simulink model "lab10"  (R2024a)
settings: Solver=VariableStepAuto  StartTime=0.0  StopTime=100  RelTol=1e-3  EnableMultiTasking=on
model workspace (MAT data in the model file):
  GGwp = 5
undefined symbols (not defined in the file): m, n
libraries: simulink x2, spsMonostableLib x1, commrandsrc3 x1
settings Model: SimulationMode=accelerator  Creator=The MathWorks, Inc.  LastModifiedBy=user
settings SolverCC: AlgebraicLoopSolver=TrustRegion
settings DataIOCC: LimitDataPoints=on  SaveFormat=Array  ReturnWorkspaceOutputs=off
settings OptimizationCC: LifeSpan=inf
settings DebuggingCC: UnconnectedInputMsg=warning  UnconnectedOutputMsg=warning  UnconnectedLineMsg=warning  AllowSymbolicDim=off  SFUnexpectedBacktrackingDiag=warning  SFNoUnconditionalDefaultTransitionDiag=warning  SFExecutionAtInitializationDiag=none  ArithmeticOperatorsInVariantConditions=warning
settings ModelReferenceCC: EnableRefExpFcnMdlSchedulingChecks=on  PropagateSignalLabelsOutOfModel=off
settings SFSimCC: SimUseLocalCustomCode=off  CustomCodeUndefinedFunction=UseInterfaceOnly
settings RTWCC: RTWUseLocalCustomCode=off  GPUComputeCapability=3.5  DLArmComputeVersion=19.05
settings CodeAppCC: StateflowObjectComments=on
settings GRTTargetCC: TargetLangStandard=C89/C90 (ANSI)
settings ConfigComp: CovMetricSettings=dw  CovSaveCumulativeToWorkspaceVar=on  CovSaveSingleToWorkspaceVar=on  CovExternalEMLEnable=off  CovSFcnEnable=off

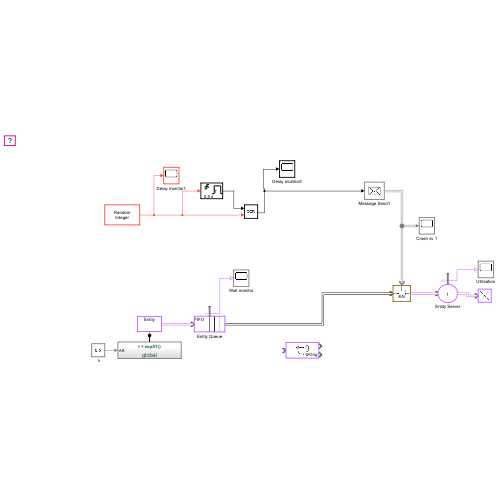
[thumbnail: Simulink's stored preview of the top-level diagram]
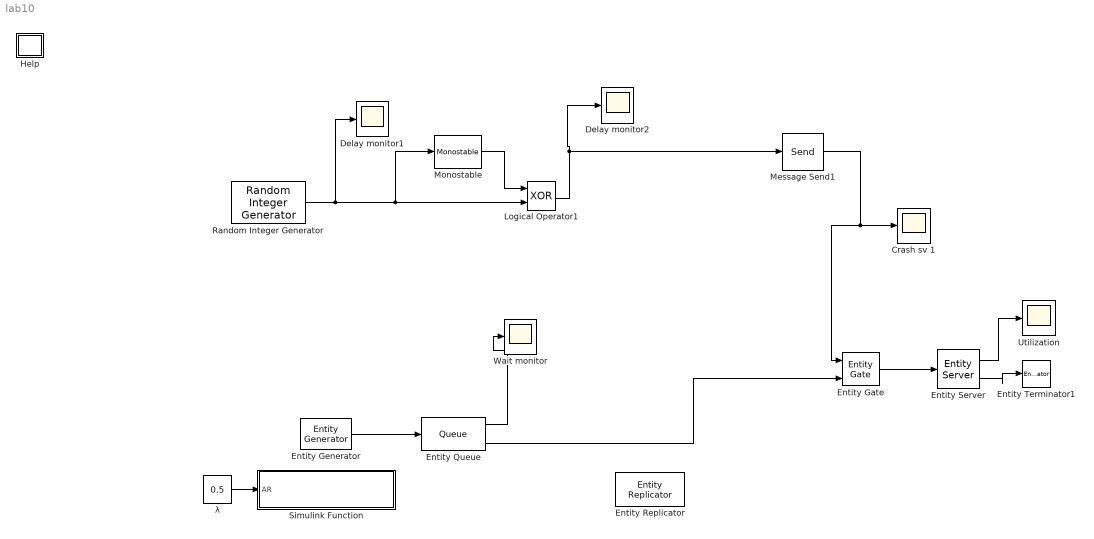
== system lab10 ==
  " λ" : Constant  Value=0.5  SampleTime=-1
  Crash sv 1 : Scope
  Delay monitor1 : Scope
  Delay monitor2 : Scope
  Entity Gate : EntityGate  InputPortMessageModes=m,m  OutputPortMessageModes=m
  Entity Generator : EntityGenerator  OutputPortMessageModes=m  TimeSource=MATLAB action  IntergenerationTimeAction=dt = expAT();  AttributeName=entity  AttributeInitialValue=0  EntityType=Structured  EntityTypeName=Entity
  Entity Queue : Queue  InputPortMessageModes=m  OutputPortMessageModes=n,m  Capacity=inf  AverageWait=on
      settings: OutputPortMap=o2,o5
  Entity Replicator : EntityReplicator  InputPortMessageModes=m  OutputPortMessageModes=m,m
  Entity Server : EntityServer  InputPortMessageModes=m  OutputPortMessageModes=n,m  Capacity=1  Utilization=on
      settings: OutputPortMap=o5,o9
  Entity Terminator1 : EntityTerminator  InputPortMessageModes=m
  Help : Subsystem
      settings: OpenFcn=showExample('simevents/MM1QueuingSysExample');
      mask Display: disp('?')
  Logical Operator1 : Logic  Operator=XOR  AllPortsSameDT=off  OutDataTypeStr=boolean
  Message Send1 : Send  OutputPortMessageModes=m
  Monostable : spsMonostableLib/Monostable  EdgeDetect=Rising  PulseDuration=0.5  ic=1  Ts=0
      settings: LibrarySourceBlock=sps_lib/Control/Monostable
  Random Integer Generator : commrandsrc3/Random Integer Generator  SetSize=2  SeedSource=Parameter  Seed=0  SampleTime=1  SamplesPerFrame=1  OutputDataType=boolean  SimulateUsing=Interpreted execution
  Simulink Function : Subsystem  TreatAsAtomicUnit=on
  Utilization : Scope
  Wait monitor : Scope
  wires:
  " λ"/1 -> Simulink Function/1(AR)
  Entity Gate/1 -> Entity Server/1
  Entity Generator/1 -> Entity Queue/1
  Message Send1/1 -> Entity Gate/1, Crash sv 1/1
  Logical Operator1/1 -> Delay monitor2/1, Message Send1/1
  Entity Queue/1 -> Wait monitor/1
  Entity Server/2 -> Entity Terminator1/1
  Random Integer Generator/1 -> Delay monitor1/1, Monostable/1, Logical Operator1/2
  Entity Server/1 -> Utilization/1
  Monostable/1 -> Logical Operator1/1
  Entity Queue/2 -> Entity Gate/2

== system lab10/Help ==

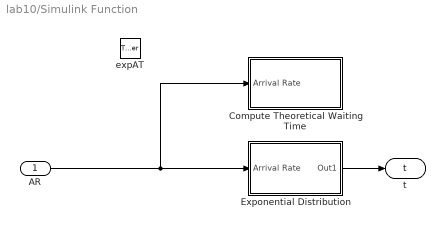
== system lab10/Simulink Function ==
  AR : Inport
  expAT : TriggerPort  TriggerType=function-call  IsSimulinkFunction=on  FunctionName=expAT  VariantControl=Variant
  Compute Theoretical Waiting Time : Subsystem
  Exponential Distribution : Subsystem
  t : ArgOut  DisableCoverage=on  ArgumentName=t
  wires:
  AR/1 -> Compute Theoretical Waiting Time/1(Arrival Rate), Exponential Distribution/1(Arrival Rate)
  Exponential Distribution/1(Out1) -> t/1

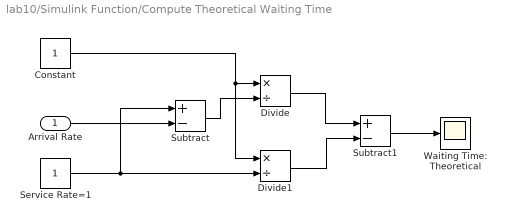
== system lab10/Simulink Function/Compute Theoretical Waiting Time ==
  Arrival Rate : Inport
  Constant : Constant
  Divide : Product  Inputs=*/
  Divide1 : Product  Inputs=*/
  Service Rate=1 : Constant
  Subtract : Sum  Inputs=+-
  Subtract1 : Sum  Inputs=+-
  Waiting Time: Theoretical : Scope
  wires:
  Arrival Rate/1 -> Subtract/2
  Subtract1/1 -> Waiting Time: Theoretical/1
  Divide1/1 -> Subtract1/2
  Divide/1 -> Subtract1/1
  Subtract/1 -> Divide/2
  Constant/1 -> Divide1/1, Divide/1
  Service Rate=1/1 -> Subtract/1, Divide1/2

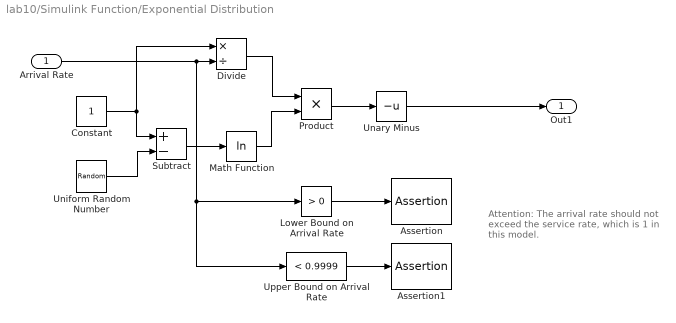
== system lab10/Simulink Function/Exponential Distribution ==
  note: Attention: The arrival rate
      | should not exceed the service
      | rate, which is 1 in this model.
  Arrival Rate : Inport
  Assertion : Assertion
  Assertion1 : Assertion
  Constant : Constant
  Divide : Product  Inputs=*/
  Lower Bound on Arrival Rate : simulink/Logic and Bit Operations/Compare To Constant  relop=>  const=0  OutDataTypeStr=uint8  ZeroCross=off
  Math Function : Math  Operator=log  SignedPower=on
  Product : Product  RndMeth=Zero
  Subtract : Sum  Inputs=+-
  Unary Minus : UnaryMinus
  Uniform Random Number : UniformRandomNumber  Minimum=0  Seed=12345
  "Upper Bound on Arrival Rate " : simulink/Logic and Bit Operations/Compare To Constant  relop=<  const=0.9999  OutDataTypeStr=uint8  ZeroCross=off
  Out1 : Outport
  wires:
  Arrival Rate/1 -> Divide/2, Lower Bound on Arrival Rate/1, "Upper Bound on Arrival Rate "/1
  Unary Minus/1 -> Out1/1
  Product/1 -> Unary Minus/1
  Math Function/1 -> Product/2
  Divide/1 -> Product/1
  Constant/1 -> Divide/1, Subtract/1
  Uniform Random Number/1 -> Subtract/2
  Lower Bound on Arrival Rate/1 -> Assertion/1
  "Upper Bound on Arrival Rate "/1 -> Assertion1/1
  Subtract/1 -> Math Function/1
